simulink model "System_Level_Behavioral"  (R2025b)
settings: Solver=VariableStepDiscrete  StartTime=0.0  StopTime=0.01  RelTol=1e-3
InitFcn:
  | fs         = 8e6;
  | Ts         = 1/fs;
  | fc         = 2.4e9;
  | c          = physconst("LightSpeed");
  | lambda     = freq2wavelen(fc,c);
  | arraySize  = [8,8];
  | targetRCS  = 10.0;
  | targetDist = 30e3;
  | pulseWidth = 1e-6;
  | PRF        = 4000;
  | maxRange   = 40e3;
  | 
  | %% Matched filter parameters
  | estimatedDelay = 0; % signal processing delay (in case of buffering)
  | 
  | hwav = phased.RectangularWaveform(...
  |     'PulseWidth',pulseWidth,...
  |     'PRF',PRF,...
  |     'SampleRate',fs);
  | matchingCoeff = getMatchedFilter(hwav);
  | % Delay introduced due to filter
  | matchingDelay = size(matchingCoeff,1)-1;
  | 
  | % Time varying gain parameters
  | fastTimeGrid = unigrid(0,1/fs,1/PRF,'[)');
  | rangeGates = c*fastTimeGrid/2;
  | metersPerSample = rangeGates(2);
  | rangeOffset = -rangeGates(2)*(matchingDelay+estimatedDelay);
  | rangeLoss = 2*fspl(rangeGates,lambda);
  | rangeLoss(1:5) = 0;
  | rangeLoss(end:end-1) = 0;
  | referenceLoss = 2*fspl(maxRange,lambda);
undefined symbols (not defined in the file): physconst
libraries: dspstat3 x8, phasedenvlib x4, phaseddetectlib x3, rfmathmodels2 x2, phasedtxrxlib x2, commrflib2 x1, simulink x1, phasedwavlib x1
settings Model: Creator=galberti  LastModifiedBy=galberti

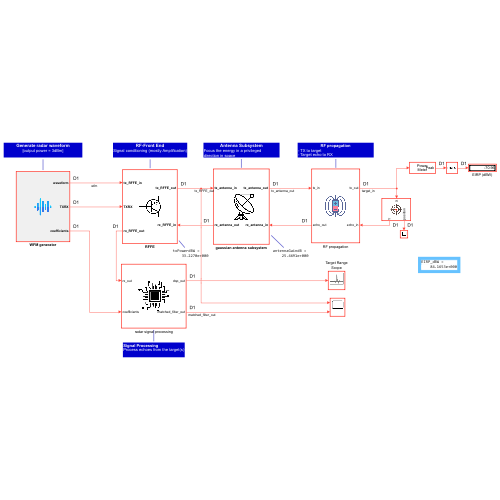
[thumbnail: Simulink's stored preview of the top-level diagram]
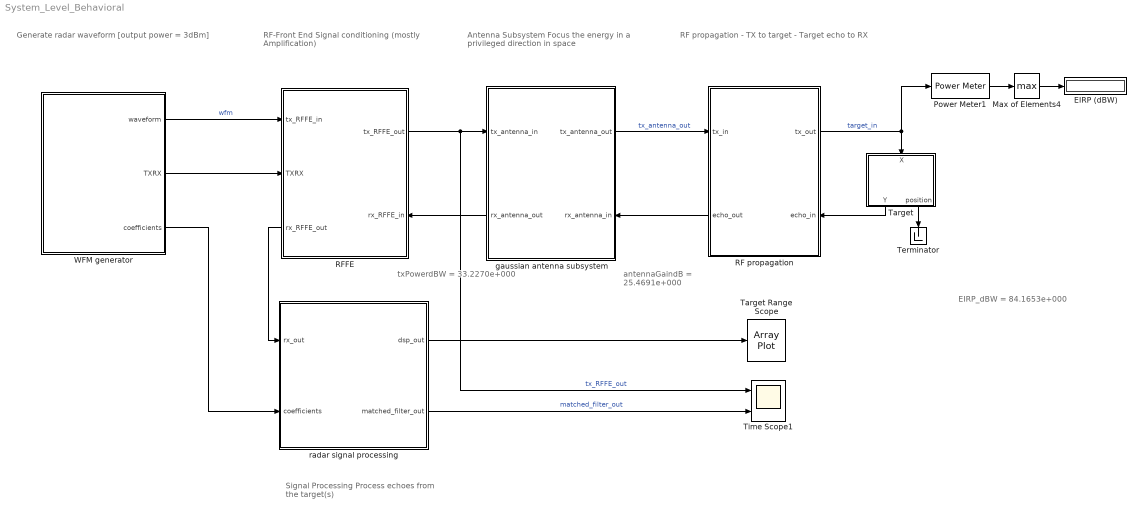
== system System_Level_Behavioral ==
  note: EIRP_dBW =
      | 84.1653e+000
  note: antennaGaindB =
      | 25.4691e+000
  note: txPowerdBW =
      | 33.2270e+000
  note: Generate radar waveform
      | [output power = 3dBm]
  note: RF-Front End
      | Signal conditioning (mostly Amplification)
  note: Antenna Subsystem
      | Focus the energy in a privileged
      | direction in space
  note: Signal Processing
      | Process echoes from the target(s)
  note: RF propagation
      | - TX to target
      | - Target echo to RX
  EIRP (dBW) : Display
  Max of Elements4 : MinMax  Function=max
  Power Meter1 : dspstat3/Power Meter  Measurement=Peak power  ReferenceLoad=1  OutputPowerUnits=dBW  WindowLength=256  OverlapLength=255  AllowArbitraryInputLength=off  ComputeCCDF=off  PowerRange=50  PowerResolution=0.1  CCDFOutput=Relative power (dB above average power)  ProbabilityVector=[ 10; 1; 0.1; 0.01; 0.001; 0.0001 ]  RelativePowerVector=[ 0; 3; 6; 9; 12 ]  ResetPort=off  SimulateUsing=Interpreted execution
  RF propagation : Subsystem
      settings: PortSchema="{\"entries\":[{\"content\":{\"sides\":[{\"content\":{\"connectorIds\":[\"In1\",\"Out2\"]},\"type\":\"ConnectorPlacement.EquallySpacedRectSide\",\"uuid\":\"4a1c7530-7650-4dc9-828c-c105decb95b0\"},{\"content\":{\"connectorIds\":[\"Out1\",\"In2\"],\"side\":\"RIGHT\"},\"type\":\"ConnectorPlacement.EquallySpacedRectSide\",\"uuid\":\"d3ec3a06-d85c-4d77-b8ee-6c5e19a3832b\"},{\"content\":{\"side\":\"TOP\"},\"type\":\"ConnectorPlacement.EquallySpacedRectSide\",\"uuid\":\"eb5f04b0-97d0-44f9-917a-0a19ff17b8bd\"}]},\"type\":\"ConnectorPlacement.EquallySpacedConnector\",\"uuid\":\"636c631f-5f34-44d2-af89-1574ca2134a6\"}],\"packageUris\":[\"http://schema.mathworks.com/mf0/Connector/R2020b\"],\"version\":\"1.0\"}"
      mask Display: image('magnet.png', [0,0,0,0,50,50]);
  RFFE : Subsystem
      settings: PortSchema="{\"entries\":[{\"content\":{\"sides\":[{\"content\":{\"connectorIds\":[\"In1\",\"In2\",\"Out2\"]},\"type\":\"ConnectorPlacement.EquallySpacedRectSide\",\"uuid\":\"4a1c7530-7650-4dc9-828c-c105decb95b0\"},{\"content\":{\"connectorIds\":[\"Out1\",\"In3\"],\"side\":\"RIGHT\"},\"type\":\"ConnectorPlacement.EquallySpacedRectSide\",\"uuid\":\"d3ec3a06-d85c-4d77-b8ee-6c5e19a3832b\"},{\"content\":{\"side\":\"TOP\"},\"type\":\"ConnectorPlacement.EquallySpacedRectSide\",\"uuid\":\"eb5f04b0-97d0-44f9-917a-0a19ff17b8bd\"},{\"content\":{\"side\":\"BOTTOM\"},\"type\":\"ConnectorPlacement.EquallySpacedRectSide\",\"uuid\":\"a4516c16-68ea-4392-9164-a0e22396dad7\"}]},\"type\":\"ConnectorPlacement.EquallySpacedConnector\",\"uuid\":\"636c631f-5f34-44d2-af89-1574ca2134a6\"}],\"packageUris\":[\"http://schema.mathworks.com/mf0/Connector/R2020b\"],\"version\":\"1.0\"}"
      mask Display: image('transistor.png', [0,0,0,0,50,50]);
  Target : Subsystem
      settings: PortSchema="{\"entries\":[{\"content\":{\"sides\":[{\"content\":{},\"type\":\"ConnectorPlacement.EquallySpacedRectSide\",\"uuid\":\"8a6fd2f7-d15e-4a2e-b1e0-7a96b21b95fb\"},{\"content\":{\"side\":\"RIGHT\"},\"type\":\"ConnectorPlacement.EquallySpacedRectSide\",\"uuid\":\"bc3a7d9e-f691-43b7-91d6-b93852d4fa00\"},{\"content\":{\"connectorIds\":[\"In1\"],\"side\":\"TOP\"},\"type\":\"ConnectorPlacement.EquallySpacedRectSide\",\"uuid\":\"7ed9c8d2-fd28-46f2-9526-28705f091796\"},{\"content\":{\"connectorIds\":[\"Out1\",\"Out2\"],\"side\":\"BOTTOM\"},\"type\":\"ConnectorPlacement.EquallySpacedRectSide\",\"uuid\":\"18e6cb2d-6873-45d3-ad7e-d642b2ec4bb6\"}]},\"type\":\"ConnectorPlacement.EquallySpacedConnector\",\"uuid\":\"97cbfb25-2a62-4885-bca6-0491b6cac52b\"}],\"packageUris\":[\"http://schema.mathworks.com/mf0/Connector/R2020b\"],\"version\":\"1.0\"}"
      mask Display: image('target.png', [0,0,0,0,50,50]);
  Target Range Scope : ArrayPlot  WindowPosition=[364.000000,22.000000,672.000000,333.000000,]  ScopeFrameLocation=window  SampleIncrement=metersPerSample  XOffset=rangeOffset  PlotType=Line  AxesScaling=Manual  MaximizeAxes=On  Title=Radar Return  XLabel=Range (m)  YLimits=[-0.000033996 0.000305962]
  Terminator : Terminator
  Time Scope1 : Scope  NumInputPorts=2
      settings: TimeUnits=Metric (based on Time Span)  PlotAsMagnitudePhase=on  ActiveDisplayYMinimum=-1.8948346455901889E-5  ActiveDisplayYMaximum=0.00017053511810311703  YLabel=Amplitude
  WFM generator : Subsystem
      mask Display: image('wave-sound.png', [0,0,0,0,32,32]);
  gaussian antenna subsystem : Subsystem
      settings: PortSchema="{\"entries\":[{\"content\":{\"sides\":[{\"content\":{\"connectorIds\":[\"In1\",\"Out2\"]},\"type\":\"ConnectorPlacement.EquallySpacedRectSide\",\"uuid\":\"4a1c7530-7650-4dc9-828c-c105decb95b0\"},{\"content\":{\"connectorIds\":[\"Out1\",\"In2\"],\"side\":\"RIGHT\"},\"type\":\"ConnectorPlacement.EquallySpacedRectSide\",\"uuid\":\"d3ec3a06-d85c-4d77-b8ee-6c5e19a3832b\"},{\"content\":{\"side\":\"TOP\"},\"type\":\"ConnectorPlacement.EquallySpacedRectSide\",\"uuid\":\"eb5f04b0-97d0-44f9-917a-0a19ff17b8bd\"},{\"content\":{\"side\":\"BOTTOM\"},\"type\":\"ConnectorPlacement.EquallySpacedRectSide\",\"uuid\":\"53210fec-ed1a-4dc4-91e9-224cfdf02ee3\"}]},\"type\":\"ConnectorPlacement.EquallySpacedConnector\",\"uuid\":\"636c631f-5f34-44d2-af89-1574ca2134a6\"}],\"packageUris\":[\"http://schema.mathworks.com/mf0/Connector/R2020b\"],\"version\":\"1.0\"}"
      mask Display: image('antenna.png', [0,0,0,0,50,50]);
  radar signal processing : Subsystem
      mask Display: image('chip.png', [0,0,0,0,50,50]);
  wires:
  WFM generator/1(waveform) -> RFFE/1(tx_RFFE_in)  "wfm"
  WFM generator/3(coefficients) -> radar signal processing/2(coefficients)
  RF propagation/1(tx_out) -> Power Meter1/1, Target/1(X)  "target_in"
  RFFE/1(tx_RFFE_out) -> Time Scope1/1, gaussian antenna subsystem/1(tx_antenna_in)  "tx_RFFE_out"
  WFM generator/2(TXRX) -> RFFE/2(TXRX)
  gaussian antenna subsystem/1(tx_antenna_out) -> RF propagation/1(tx_in)  "tx_antenna_out"
  gaussian antenna subsystem/2(rx_antenna_out) -> RFFE/3(rx_RFFE_in)
  RFFE/2(rx_RFFE_out) -> radar signal processing/1(rx_out)
  RF propagation/2(echo_out) -> gaussian antenna subsystem/2(rx_antenna_in)
  radar signal processing/1(dsp_out) -> Target Range Scope/1
  radar signal processing/2(matched_filter_out) -> Time Scope1/2  "matched_filter_out"
  Power Meter1/1 -> Max of Elements4/1
  Max of Elements4/1 -> EIRP (dBW)/1
  Target/1(Y) -> RF propagation/2(echo_in)
  Target/2(position) -> Terminator/1

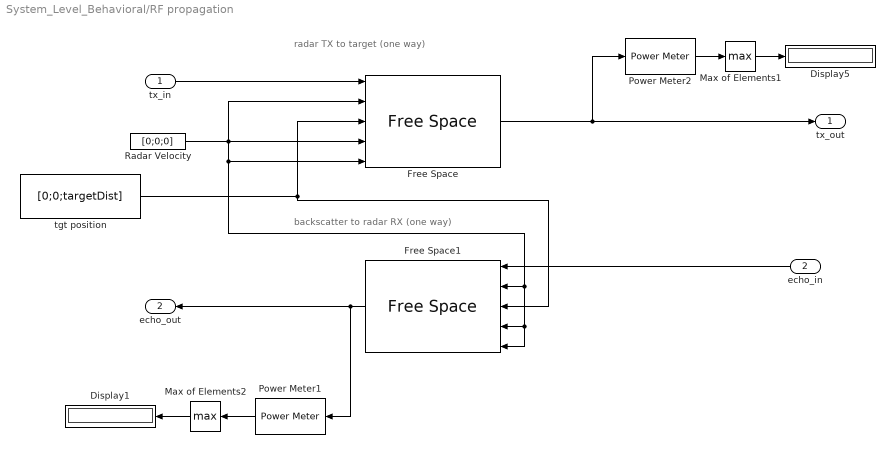
== system System_Level_Behavioral/RF propagation ==
  note: backscatter to radar RX (one way)
  note: radar TX to target (one way)
  tx_in : Inport
  echo_in : Inport  Port=2
  Display1 : Display
  Display5 : Display
  Free Space : phasedenvlib/Free Space  PropagationSpeed=physconst( 'LightSpeed' )  OperatingFrequency=fc  TwoWayPropagation=off  SampleRateFromInputCheckbox=off  SampleRate=fs  MaximumDistanceSource=Property  MaximumDistance=2*max(targetDist)  MaximumNumInputSamplesSource=Auto  MaximumNumInputSamples=1000  SimulateUsing=Interpreted execution
  Free Space1 : phasedenvlib/Free Space  PropagationSpeed=physconst( 'LightSpeed' )  OperatingFrequency=fc  TwoWayPropagation=off  SampleRateFromInputCheckbox=on  SampleRate=1e6  MaximumDistanceSource=Property  MaximumDistance=2*max(targetDist)  MaximumNumInputSamplesSource=Auto  MaximumNumInputSamples=1000  SimulateUsing=Interpreted execution
  Max of Elements1 : MinMax  Function=max
  Max of Elements2 : MinMax  Function=max
  Power Meter1 : dspstat3/Power Meter  Measurement=Peak power  ReferenceLoad=1  OutputPowerUnits=dBW  WindowLength=256  OverlapLength=255  AllowArbitraryInputLength=off  ComputeCCDF=off  PowerRange=50  PowerResolution=0.1  CCDFOutput=Relative power (dB above average power)  ProbabilityVector=[ 10; 1; 0.1; 0.01; 0.001; 0.0001 ]  RelativePowerVector=[ 0; 3; 6; 9; 12 ]  ResetPort=off  SimulateUsing=Interpreted execution
  Power Meter2 : dspstat3/Power Meter  Measurement=Peak power  ReferenceLoad=1  OutputPowerUnits=dBW  WindowLength=256  OverlapLength=255  AllowArbitraryInputLength=off  ComputeCCDF=off  PowerRange=50  PowerResolution=0.1  CCDFOutput=Relative power (dB above average power)  ProbabilityVector=[ 10; 1; 0.1; 0.01; 0.001; 0.0001 ]  RelativePowerVector=[ 0; 3; 6; 9; 12 ]  ResetPort=off  SimulateUsing=Interpreted execution
  Radar Velocity : Constant  Value=[0;0;0]  SampleTime=-1
  tgt position : Constant  Value=[0;0;targetDist]  SampleTime=-1
  tx_out : Outport
  echo_out : Outport  Port=2
  wires:
  tx_in/1 -> Free Space/1
  Free Space1/1 -> echo_out/1, Power Meter1/1
  Free Space/1 -> Power Meter2/1, tx_out/1
  echo_in/1 -> Free Space1/1
  Radar Velocity/1 -> Free Space/5, Free Space1/5, Free Space1/4, Free Space1/2, Free Space/2, Free Space/4
  tgt position/1 -> Free Space/3, Free Space1/3
  Power Meter2/1 -> Max of Elements1/1
  Max of Elements1/1 -> Display5/1
  Power Meter1/1 -> Max of Elements2/1
  Max of Elements2/1 -> Display1/1

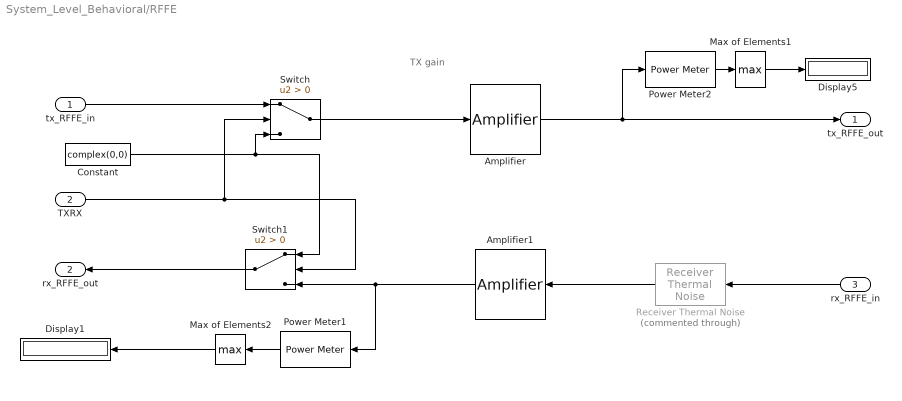
== system System_Level_Behavioral/RFFE ==
  note: TX gain
  tx_RFFE_in : Inport
  TXRX : Inport  Port=2
  rx_RFFE_in : Inport  Port=3
  Amplifier : rfmathmodels2/Amplifier  Model=cubic  Gain=60  Nonlinearity=OIP3  IIP3=Inf  OIP3=Inf  IP1dB=Inf  OP1dB=Inf  IPsat=Inf  OPsat=Inf  Table=[ -25, 5, -1; -10, 20, -2; 0, 27, 5; 5, 28, 12 ]  MagnitudeGainDB=0  Vsat=1  MagnitudeSmooth=2  PhaseGainRadian=-.45  PhaseSaturation=.88  PhaseSmooth=[ 3.43, 3.43 ]  InputScaleDB=0  AmAmParameters=[ 2.1587, 1.1517 ]  AmPmParameters=[ 4.0033, 9.1040 ]  OutputScaleDB=0  SimulateUsing=Interpreted execution  IncludeNoise=off  NoiseType=NF  NoiseTemperature=290  NF=3  NoiseFactor=2  SeedSource=auto  Seed=67987  SampleRate=1e6
  Amplifier1 : rfmathmodels2/Amplifier  Model=cubic  Gain=39  Nonlinearity=OIP3  IIP3=Inf  OIP3=Inf  IP1dB=Inf  OP1dB=Inf  IPsat=Inf  OPsat=Inf  Table=[ -25, 5, -1; -10, 20, -2; 0, 27, 5; 5, 28, 12 ]  MagnitudeGainDB=0  Vsat=1  MagnitudeSmooth=2  PhaseGainRadian=-.45  PhaseSaturation=.88  PhaseSmooth=[ 3.43, 3.43 ]  InputScaleDB=0  AmAmParameters=[ 2.1587, 1.1517 ]  AmPmParameters=[ 4.0033, 9.1040 ]  OutputScaleDB=0  SimulateUsing=Interpreted execution  IncludeNoise=off  NoiseType=NF  NoiseTemperature=290  NF=6  NoiseFactor=2  SeedSource=auto  Seed=67987  SampleRate=1e6
  Constant : Constant  Value=complex(0,0)  OutDataTypeStr=Inherit: Inherit via back propagation
  Display1 : Display
  Display5 : Display
  Max of Elements1 : MinMax  Function=max
  Max of Elements2 : MinMax  Function=max
  Power Meter1 : dspstat3/Power Meter  Measurement=Peak power  ReferenceLoad=1  OutputPowerUnits=dBW  WindowLength=256  OverlapLength=255  AllowArbitraryInputLength=off  ComputeCCDF=off  PowerRange=50  PowerResolution=0.1  CCDFOutput=Relative power (dB above average power)  ProbabilityVector=[ 10; 1; 0.1; 0.01; 0.001; 0.0001 ]  RelativePowerVector=[ 0; 3; 6; 9; 12 ]  ResetPort=off  SimulateUsing=Interpreted execution
  Power Meter2 : dspstat3/Power Meter  Measurement=Peak power  ReferenceLoad=1  OutputPowerUnits=dBW  WindowLength=256  OverlapLength=255  AllowArbitraryInputLength=off  ComputeCCDF=off  PowerRange=50  PowerResolution=0.1  CCDFOutput=Relative power (dB above average power)  ProbabilityVector=[ 10; 1; 0.1; 0.01; 0.001; 0.0001 ]  RelativePowerVector=[ 0; 3; 6; 9; 12 ]  ResetPort=off  SimulateUsing=Interpreted execution
  Receiver Thermal Noise : commrflib2/Receiver Thermal Noise  Commented=through  LegacyMode=off  NoiseMethod=Noise temperature  NoiseTemperature=290  NoiseFigure=3.0103  NoiseFactor=2  Add290KAntennaNoise=off  ReferenceLoad=1  RandomStream=Global stream  Seed=floor(rand(1,1)*1000)  SimulateUsing=Interpreted execution
  Switch : Switch  Criteria=u2 > Threshold  SaturateOnIntegerOverflow=off  InputSameDT=off
  Switch1 : Switch  Criteria=u2 > Threshold  SaturateOnIntegerOverflow=off  InputSameDT=off
  tx_RFFE_out : Outport
  rx_RFFE_out : Outport  Port=2
  wires:
  tx_RFFE_in/1 -> Switch/1
  Amplifier/1 -> Power Meter2/1, tx_RFFE_out/1
  Switch/1 -> Amplifier/1
  Constant/1 -> Switch1/1, Switch/3
  Receiver Thermal Noise/1 -> Amplifier1/1
  rx_RFFE_in/1 -> Receiver Thermal Noise/1
  Amplifier1/1 -> Power Meter1/1, Switch1/3
  Switch1/1 -> rx_RFFE_out/1
  TXRX/1 -> Switch1/2, Switch/2
  Power Meter2/1 -> Max of Elements1/1
  Max of Elements1/1 -> Display5/1
  Power Meter1/1 -> Max of Elements2/1
  Max of Elements2/1 -> Display1/1

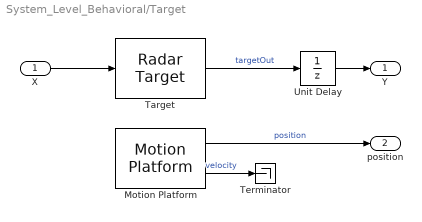
== system System_Level_Behavioral/Target ==
  X : Inport
  Motion Platform : phasedenvlib/Motion Platform  MotionModel=Velocity  InitialPosition=[0;0;30e3]  InitialVelocity=[ 0; 0; 0 ]  VelocitySource=Property  Velocity=[0;0;0]  AccelerationSource=Property  Acceleration=[0;0;0]  CustomTrajectory=[ 0, 0, 0, 0, 0, 0, 0; 1, 0, 0, 0, 0, 0, 0 ]  ScanMode=None  InitialScanAngle=0  AzimuthSpan=[ -60, 60 ]  AzimuthScanRate=10  InitialOrientationAxes=eye(3)  OrientationAxesOutputPort=off  ElapsedTimeSource=Auto  SampleRateFromInputCheckbox=on  SampleRate=1e6  SimulateUsing=Interpreted execution
  Target : phasedenvlib/Radar Target  EnablePolarization=off  Mode=Monostatic  MeanRCSSource=Property  ScatteringMatrixSource=Property  MeanRCS=targetRCS  ScatteringMatrix=eye( 2 )  Model=Nonfluctuating  PropagationSpeed=physconst('LightSpeed')  OperatingFrequency=fc  SeedSource=Auto  Seed=0  SimulateUsing=Interpreted execution
  Terminator : Terminator
  Unit Delay : UnitDelay  SampleTime=-1  HasFrameUpgradeWarning=on
  Y : Outport  VectorParamsAs1DForOutWhenUnconnected=off
  position : Outport  Port=2  VectorParamsAs1DForOutWhenUnconnected=off
  wires:
  X/1 -> Target/1
  Target/1 -> Unit Delay/1  "targetOut"
  Motion Platform/1 -> position/1  "position"
  Motion Platform/2 -> Terminator/1  "velocity"
  Unit Delay/1 -> Y/1

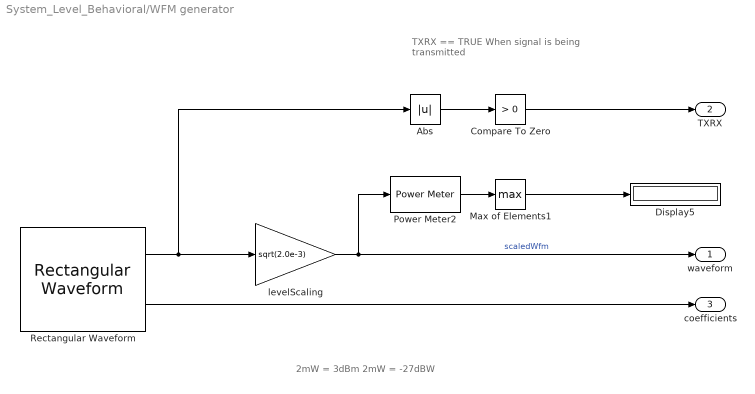
== system System_Level_Behavioral/WFM generator ==
  note: 2mW = 3dBm
      | 2mW = -27dBW
  note: TXRX == TRUE
      | When signal is being transmitted
  Abs : Abs  SaturateOnIntegerOverflow=off
  Compare To Zero : simulink/Logic and Bit Operations/Compare To Zero  relop=>  OutDataTypeStr=boolean
  Display5 : Display
  Max of Elements1 : MinMax  Function=max
  Power Meter2 : dspstat3/Power Meter  Measurement=Peak power  ReferenceLoad=1  OutputPowerUnits=dBW  WindowLength=256  OverlapLength=255  AllowArbitraryInputLength=off  ComputeCCDF=off  PowerRange=50  PowerResolution=0.1  CCDFOutput=Relative power (dB above average power)  ProbabilityVector=[ 10; 1; 0.1; 0.01; 0.001; 0.0001 ]  RelativePowerVector=[ 0; 3; 6; 9; 12 ]  ResetPort=off  SimulateUsing=Interpreted execution
  Rectangular Waveform : phasedwavlib/Rectangular Waveform  SampleRate=fs  DurationSpecification=Pulse width  PulseWidth=pulseWidth  DutyCycle=0.5  PRF=PRF  PRFSelectionInputPort=off  SimulationTimeSource=Derive from waveform parameters  FrequencyOffsetSource=Property  FrequencyOffset=0  OutputFormat=Pulses  NumSamples=100  NumPulses=1  PRFOutputPort=off  CoefficientsOutputPort=on  SimulateUsing=Interpreted execution
  levelScaling : Gain  Gain=sqrt(2.0e-3)
  waveform : Outport
  TXRX : Outport  Port=2
  coefficients : Outport  Port=3
  wires:
  Rectangular Waveform/2 -> coefficients/1
  Rectangular Waveform/1 -> Abs/1, levelScaling/1
  levelScaling/1 -> Power Meter2/1, waveform/1  "scaledWfm"
  Abs/1 -> Compare To Zero/1
  Compare To Zero/1 -> TXRX/1
  Power Meter2/1 -> Max of Elements1/1
  Max of Elements1/1 -> Display5/1

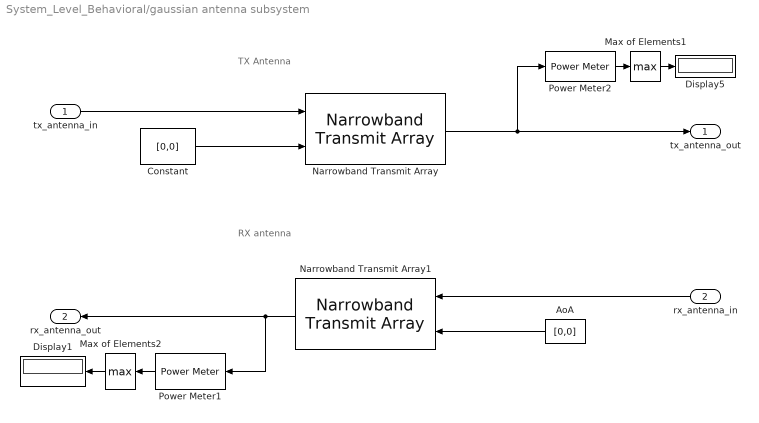
== system System_Level_Behavioral/gaussian antenna subsystem ==
  note: RX antenna
  note: TX Antenna
  tx_antenna_in : Inport
  rx_antenna_in : Inport  Port=2
  AoA : Constant  Value=[0,0]
  Constant : Constant  Value=[0,0]
  Display1 : Display
  Display5 : Display
  Max of Elements1 : MinMax  Function=max
  Max of Elements2 : MinMax  Function=max
  Narrowband Transmit Array : phasedtxrxlib/Narrowband Transmit Array  PropagationSpeed=physconst( 'LightSpeed' )  OperatingFrequency=fc  CombineRadiatedSignals=on  SensorGainMeasure=dBi  Polarization=None  WeightsInputPort=off  SimulateUsing=Interpreted execution  Sensor=phased.GaussianAntennaElement(Beamwidth=[ 10, 10 ])
  Narrowband Transmit Array1 : phasedtxrxlib/Narrowband Transmit Array  PropagationSpeed=physconst( 'LightSpeed' )  OperatingFrequency=fc  CombineRadiatedSignals=on  SensorGainMeasure=dBi  Polarization=None  WeightsInputPort=off  SimulateUsing=Interpreted execution  Sensor=phased.GaussianAntennaElement(Beamwidth=[ 10, 10 ])
  Power Meter1 : dspstat3/Power Meter  Measurement=Peak power  ReferenceLoad=1  OutputPowerUnits=dBW  WindowLength=256  OverlapLength=255  AllowArbitraryInputLength=off  ComputeCCDF=off  PowerRange=50  PowerResolution=0.1  CCDFOutput=Relative power (dB above average power)  ProbabilityVector=[ 10; 1; 0.1; 0.01; 0.001; 0.0001 ]  RelativePowerVector=[ 0; 3; 6; 9; 12 ]  ResetPort=off  SimulateUsing=Interpreted execution
  Power Meter2 : dspstat3/Power Meter  Measurement=Peak power  ReferenceLoad=1  OutputPowerUnits=dBW  WindowLength=256  OverlapLength=255  AllowArbitraryInputLength=off  ComputeCCDF=off  PowerRange=50  PowerResolution=0.1  CCDFOutput=Relative power (dB above average power)  ProbabilityVector=[ 10; 1; 0.1; 0.01; 0.001; 0.0001 ]  RelativePowerVector=[ 0; 3; 6; 9; 12 ]  ResetPort=off  SimulateUsing=Interpreted execution
  tx_antenna_out : Outport
  rx_antenna_out : Outport  Port=2
  wires:
  Constant/1 -> Narrowband Transmit Array/2
  Narrowband Transmit Array1/1 -> Power Meter1/1, rx_antenna_out/1
  rx_antenna_in/1 -> Narrowband Transmit Array1/1
  Narrowband Transmit Array/1 -> Power Meter2/1, tx_antenna_out/1
  AoA/1 -> Narrowband Transmit Array1/2
  tx_antenna_in/1 -> Narrowband Transmit Array/1
  Power Meter2/1 -> Max of Elements1/1
  Max of Elements1/1 -> Display5/1
  Power Meter1/1 -> Max of Elements2/1
  Max of Elements2/1 -> Display1/1

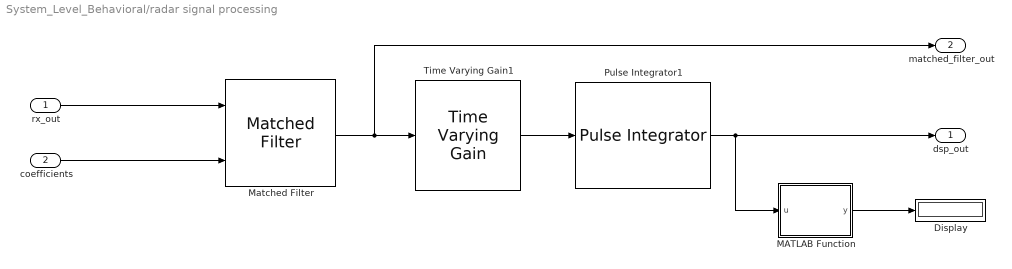
== system System_Level_Behavioral/radar signal processing ==
  rx_out : Inport
  coefficients : Inport  Port=2
  Display : Display
  MATLAB Function : MATLAB Function  TreatAsAtomicUnit=on
  Matched Filter : phaseddetectlib/Matched Filter  CoefficientsSource=Input port  Coefficients=[ 1; 1 ]  SpectrumWindow=None  CustomSpectrumWindow=@hamming  SpectrumRange=[ 0, 1e5 ]  SampleRateFromInputCheckbox=on  SampleRate=1e6  SidelobeAttenuation=30  Beta=0.5  Nbar=4  GainOutputPort=off  MaximumNumInputSamplesSource=Auto  MaximumNumInputSamples=100  SimulateUsing=Interpreted execution
  Pulse Integrator1 : phaseddetectlib/Pulse Integrator  CoherentFlag=Noncoherent  N=10  V=9
  Time Varying Gain1 : phaseddetectlib/Time Varying Gain  RangeLossSource=Property  RangeLoss=rangeLoss  ReferenceLoss=referenceLoss  SimulateUsing=Interpreted execution
  dsp_out : Outport
  matched_filter_out : Outport  Port=2
  wires:
  rx_out/1 -> Matched Filter/1
  Pulse Integrator1/1 -> MATLAB Function/1(u), dsp_out/1
  Matched Filter/1 -> matched_filter_out/1, Time Varying Gain1/1
  Time Varying Gain1/1 -> Pulse Integrator1/1
  coefficients/1 -> Matched Filter/2
  MATLAB Function/1(y) -> Display/1

== matlab function System_Level_Behavioral/radar signal processing/MATLAB Function ==
  data: u input; y output; metersPerSample parameter; rangeOffset parameter
function y = targetDistance(u, metersPerSample, rangeOffset)
[~,idx] = max(u);
N=length(u);
distance = (0:N-1)*metersPerSample+rangeOffset;
y = distance(idx)/1e3;
